simulink model "View_Speed"  (R2024b)
settings: Solver=FixedStepDiscrete  StartTime=0.0  StopTime=10.0  FixedStep=0.1  RelTol=1e-3  EnableMultiTasking=on
values from neighbouring files (symbols this model uses):
  C_BLANK = mpt.Parameter    [View_Speed_dd.m]
  C_CANADA = mpt.Parameter    [View_Speed_dd.m]
  C_DEFAULT_TOLER_A_VALUE = mpt.Parameter    [View_Speed_dd.m]
  C_DEFAULT_TOLER_B_VALUE = mpt.Parameter    [View_Speed_dd.m]
  C_MET_SPD_MAX_VALUE = mpt.Parameter    [View_Speed_dd.m]
  C_MET_SPD_MIN_THRESHOLD = mpt.Parameter    [View_Speed_dd.m]
  C_MEXICO = mpt.Parameter    [View_Speed_dd.m]
  C_SPEED_1KMPH = mpt.Parameter    [View_Speed_dd.m]
  C_SPEED_2KMPH = mpt.Parameter    [View_Speed_dd.m]
  C_SPEED_ZERO = mpt.Parameter    [View_Speed_dd.m]
  C_USA = mpt.Parameter    [View_Speed_dd.m]
  cFACTOR = mpt.Parameter    [View_Speed_dd.m]
  cOFFSET = mpt.Parameter    [View_Speed_dd.m]
  eTOLER_AOut = mpt.Parameter    [View_Speed_dd.m]
  eTOLER_BOut = mpt.Parameter    [View_Speed_dd.m]
  IGN_TRAN_TIMER_MS = mpt.Parameter    [View_Speed_dd.m]
  RESOLUTION_100 = mpt.Parameter    [View_Speed_dd.m]
  RTE_E_MAX_AGE_EXCEEDED = mpt.Parameter    [View_Speed_rte_types.m]
  RTE_E_NEVER_RECEIVED = mpt.Parameter    [View_Speed_rte_types.m]
  VAL_ONE = mpt.Parameter    [View_Speed_dd.m]
  View_Speed_cTaskPeriod = mpt.Parameter    [View_Speed_rte_types.m]
undefined symbols (not defined in the file or in its folder): Arr_u8_100_type_instance, Arr_u8_1024_type_instance, Arr_u8_10_type_instance, Arr_u8_128_type_instance, Arr_u8_16_type_instance, Arr_u8_17_type_instance, Arr_u8_2048_type_instance, Arr_u8_256_type_instance, Arr_u8_32_type_instance, Arr_u8_3_type_instance, Arr_u8_46_type_instance, Arr_u8_48_type_instance, Arr_u8_61_type_instance, Arr_u8_64_type_instance, Arr_u8_8_type_instance, Arr_u8_9_type_instance, CLUSTER_INACTIVE, eMET_SPDOut, eSP_ADR, eSP_CANADA, eSP_ECE, eSP_EUROPE, eSP_KOREA_FMVSS, eSP_KOREA_UN_R, eSP_MEXICO_FMVSS, eSP_MEXICO_UN_R, eSP_UK, eSP_USA, eVehicleSpeedABSIn, IgnOff, IgnOn, pJustRcvdStatus, RxCan_SignalClearJustRcvdStatus, RxCan_SignalGetJustRcvdStatus, RxCan_SignalInvalidProcessingControl, RxCan_SignalMissingProcessingControl, RxCan_SignalNRProcessingControl, SignalId, Status, tRxSignalId_type_instance, tRxSignalJustRcvdStatus_type_instance, tRxSignalStatus_type_instance, tTxSigConfirmStatus_type_instance, tTxSignalId_type_instance, TxCan_ClearCanSignalTxConfirmation
libraries: simulink x8
(part 2 of 2)

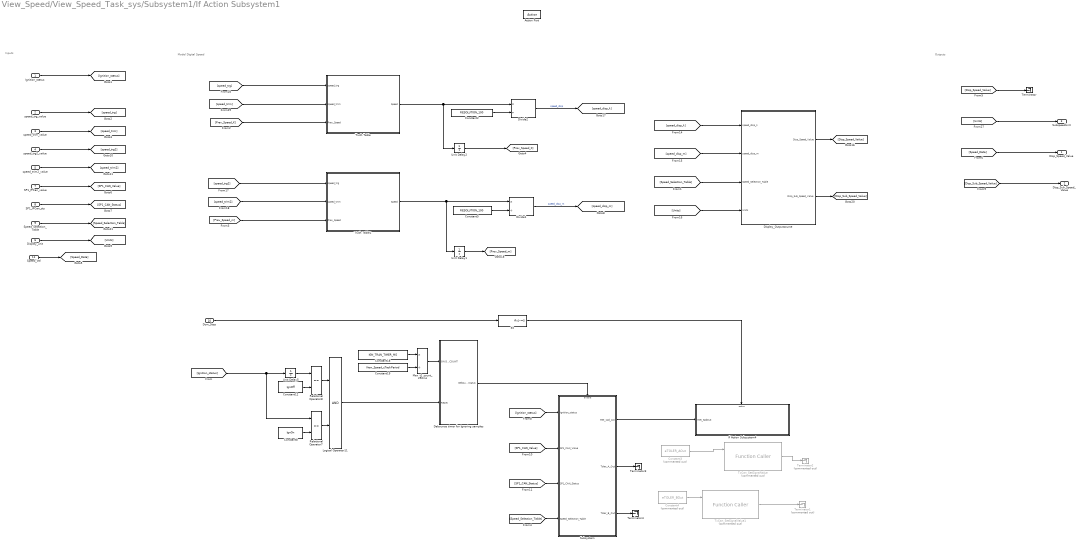
== system View_Speed/View_Speed_Task_sys/Subsystem1/If Action Subsystem1 ==
  note: Model Digital Speed
  note: Outputs
  note: Inputs
  Ignition_status : Inport  OutDataTypeStr=IgntionSubstateType
  speed_trg_value : Inport  Port=2  OutDataTypeStr=uint16
  speed_trim_value : Inport  Port=3  OutDataTypeStr=uint16
  speed_trg2_value : Inport  Port=4  OutDataTypeStr=uint16
  speed_trim2_value : Inport  Port=5  OutDataTypeStr=uint16
  Display_unit : Inport  Port=6  OutDataTypeStr=uint8
  SP1_IPCan_value : Inport  Port=7  OutDataTypeStr=uint16
  SP1_IPCan_sts : Inport  Port=8  OutDataTypeStr=uint8
  Speed_Selection_Table : Inport  Port=9  OutDataTypeStr=uint8
  Dcm_Stop : Inport  Port=10
  Speed_Val : Inport  Port=11  OutDataTypeStr=uint16
  Action Port : ActionPort  ActionPortLabel=if(u1 ~= u2)
  Constant12 : Constant  Value=IgnOff  OutDataTypeStr=uint8
  Constant18 : Constant  Value=IGN_TRAN_TIMER_MS  OutDataTypeStr=uint16
  Constant19 : Constant  Value=View_Speed_cTaskPeriod
  Constant2 : Constant  Value=RESOLUTION_100  OutDataTypeStr=uint16
  Constant3 : Constant  Commented=on  Value=eTOLER_AOut  OutDataTypeStr=uint8
  Constant4 : Constant  Commented=on  Value=eTOLER_BOut  OutDataTypeStr=uint8
  Constant5 : Constant  Value=RESOLUTION_100  OutDataTypeStr=uint16
  Constant8 : Constant  Value=IgnOn  OutDataTypeStr=uint8
  Debounce timer for Ignoring samples : Subsystem  TreatAsAtomicUnit=on
  Display_Outputsource : Subsystem
  Divide1 : Product  Inputs=*/
  Divide2 : Product  Inputs=*/
  If Action Subsystem4 : Subsystem  TreatAsAtomicUnit=on
  If2 : If  IfExpression=u1~=1  ShowElse=off
  Logical Operator11 : Logic  AllPortsSameDT=off  OutDataTypeStr=boolean
  Max_t1_count_250ms : Product  Inputs=*/  OutDataTypeStr=uint16
  Relational Operator7 : RelationalOperator  Operator===  OutDataTypeStr=boolean  InputSameDT=off
  Relational Operator8 : RelationalOperator  Operator===  OutDataTypeStr=boolean  InputSameDT=off
  Subsystem : Subsystem
  Terminator : Terminator
  Terminator1 : Terminator  Commented=on
  Terminator2 : Terminator  Commented=on
  Terminator3 : Terminator
  Terminator4 : Terminator
  Truth Table : Truth Table  TreatAsAtomicUnit=on  RTWFcnName=Speed_Value_Update
      settings: RTWSystemCode=Reusable function  RTWFcnNameOpts=User specified
  Truth Table1 : Truth Table  TreatAsAtomicUnit=on  RTWFcnName=Speed_Value_Update
      settings: RTWSystemCode=Reusable function  RTWFcnNameOpts=User specified
  TxCan_SetSignalValue : FunctionCaller  Commented=on  FunctionPrototype=error_status = TxCan_SetSignalValue(SignalId,pTxSignalData)  InputArgumentSpecifications=tTxSignalId_type_instance(1) ,uint8(1)  OutputArgumentSpecifications=uint8(1)
  TxCan_SetSignalValue1 : FunctionCaller  Commented=on  FunctionPrototype=error_status = TxCan_SetSignalValue(SignalId,pTxSignalData)  InputArgumentSpecifications=tTxSignalId_type_instance(1) ,uint8(1)  OutputArgumentSpecifications=uint8(1)
  Unit Delay1 : UnitDelay  SampleTime=-1  StateName=Prev_Speed_m  HasFrameUpgradeWarning=on
  Unit Delay2 : UnitDelay  SampleTime=-1  StateName=Prev_Speed_k  HasFrameUpgradeWarning=on
  Unit Delay5 : UnitDelay  SampleTime=-1  StateName=PrevWUSIgnState1  HasFrameUpgradeWarning=on
  Disp_Speed_Value : Outport  VectorParamsAs1DForOutWhenUnconnected=off
  Disp_Sub_Speed_Value : Outport  Port=2  VectorParamsAs1DForOutWhenUnconnected=off
  SubspeedUnit : Outport  Port=3  VectorParamsAs1DForOutWhenUnconnected=off
  wires:
  speed_trg2_value/1 -> [speed_trg2]
  SP1_IPCan_sts/1 -> [SP1_CAN_Status]
  Debounce timer for Ignoring samples/1(Debounced SW status) -> Subsystem/Enable
  speed_trim_value/1 -> [speed_trim]
  Ignition_status/1 -> [Ignition_status]
  Logical Operator11/1 -> Debounce timer for Ignoring samples/2("Reset ")
  Unit Delay5/1 -> Relational Operator8/1
  If2/1 -> If Action Subsystem4/Action
  Constant5/1 -> Divide1/2
  Max_t1_count_250ms/1 -> Debounce timer for Ignoring samples/1(ON DBNC COUNT)
  Constant12/1 -> Relational Operator8/2
  Constant18/1 -> Max_t1_count_250ms/1
  [Ignition_status] -> Subsystem/1(Ignition_status)
  [Ignition_status] -> Unit Delay5/1, Relational Operator7/1
  speed_trg_value/1 -> [speed_trg]
  [speed_disp_m] -> Display_Outputsource/2(speed_disp_m)
  Truth Table1/1(Speed) -> Unit Delay1/1, Divide1/1
  Display_unit/1 -> [Units]
  Constant19/1 -> Max_t1_count_250ms/2
  Subsystem/1(Met_spd_out) -> If Action Subsystem4/1(Met_SpdOut)
  [SP1_CAN_Value] -> Subsystem/2(SP1_CAN_Value)
  [SP1_CAN_Status] -> Subsystem/3(SP1_CAN_Status)
  Dcm_Stop/1 -> If2/1
  [speed_disp_k] -> Display_Outputsource/1(speed_disp_k)
  Relational Operator8/1 -> Logical Operator11/1
  Relational Operator7/1 -> Logical Operator11/2
  [Units] -> Display_Outputsource/4(Units)
  Constant3/1 -> TxCan_SetSignalValue/1
  Divide1/1 -> [speed_disp_m]  "speed_disp_m"
  Constant8/1 -> Relational Operator7/2
  SP1_IPCan_value/1 -> [SP1_CAN_Value]
  speed_trim2_value/1 -> [speed_trim2]
  Constant4/1 -> TxCan_SetSignalValue1/1
  [Units] -> SubspeedUnit/1
  [speed_trg] -> Truth Table/1(speed_trg)
  [speed_trim] -> Truth Table/2(speed_trim)
  Divide2/1 -> [speed_disp_k]  "speed_disp"
  Truth Table/1(Speed) -> Divide2/1, Unit Delay2/1
  Constant2/1 -> Divide2/2
  Unit Delay2/1 -> [Prev_Speed_K]
  [Prev_Speed_K] -> Truth Table/3(Prev_Speed)
  [speed_trg2] -> Truth Table1/1(speed_trg)
  [speed_trim2] -> Truth Table1/2(speed_trim)
  Unit Delay1/1 -> [Prev_Speed_m]
  [Prev_Speed_m] -> Truth Table1/3(Prev_Speed)
  Display_Outputsource/1(Disp_Speed_Value) -> [Disp_Speed_Value]
  Display_Outputsource/2(Disp_Sub_Speed_Value) -> [Disp_Sub_Speed_Value]
  [Speed_Data] -> Disp_Speed_Value/1
  [Disp_Sub_Speed_Value] -> Disp_Sub_Speed_Value/1
  Speed_Selection_Table/1 -> [Speed_Selection_Table]
  [Speed_Selection_Table] -> Display_Outputsource/3(Speed_Selection_Table)
  [Speed_Selection_Table] -> Subsystem/4(Speed_Selection_Table)
  Speed_Val/1 -> [Speed_Data]
  [Disp_Speed_Value] -> Terminator/1
  TxCan_SetSignalValue1/1 -> Terminator1/1
  TxCan_SetSignalValue/1 -> Terminator2/1
  Subsystem/2(Toler_A_Out) -> Terminator3/1
  Subsystem/3(Toler_B_Out) -> Terminator4/1

== system View_Speed/View_Speed_Task_sys/Subsystem1/If Action Subsystem1/Debounce timer for Ignoring samples ==
  note: 1. When Reset input is FALSE, allow counter to increment.
      |        (Limit to MAX when MAX count is reached)
  ON DBNC COUNT : Inport  OutDataTypeStr=uint16
  "Reset " : Inport  Port=2  OutDataTypeStr=boolean
  Constant1 : Constant  OutDataTypeStr=uint8
  Constant2 : Constant  Value=0  OutDataTypeStr=uint8
  Constant7 : Constant  Value=0  OutDataTypeStr=uint8
  Relational Operator1 : RelationalOperator  Operator=~=  OutDataTypeStr=boolean  InputSameDT=off
  Relational Operator4 : RelationalOperator  OutDataTypeStr=boolean  InputSameDT=off
  Sum : Sum  Inputs=|++
  Switch2 : Switch  Criteria=u2 ~= 0  OutDataTypeStr=uint32  SaturateOnIntegerOverflow=off  InputSameDT=off
  Switch3 : Switch  Criteria=u2 ~= 0  OutDataTypeStr=uint32  SaturateOnIntegerOverflow=off  InputSameDT=off
  Unit Delay2 : UnitDelay  SampleTime=-1  StateName=Igntran_timer_count  HasFrameUpgradeWarning=on
  Debounced SW status : Outport  VectorParamsAs1DForOutWhenUnconnected=off
  wires:
  "Reset "/1 -> Relational Operator1/2
  Constant7/1 -> Relational Operator1/1
  Relational Operator1/1 -> Switch2/2
  Switch2/1 -> Switch3/3, Relational Operator4/1
  ON DBNC COUNT/1 -> Relational Operator4/2, Switch3/1
  Switch3/1 -> Unit Delay2/1
  Constant2/1 -> Switch2/1
  Sum/1 -> Switch2/3
  Unit Delay2/1 -> Sum/2
  Constant1/1 -> Sum/1
  Relational Operator4/1 -> Debounced SW status/1, Switch3/2

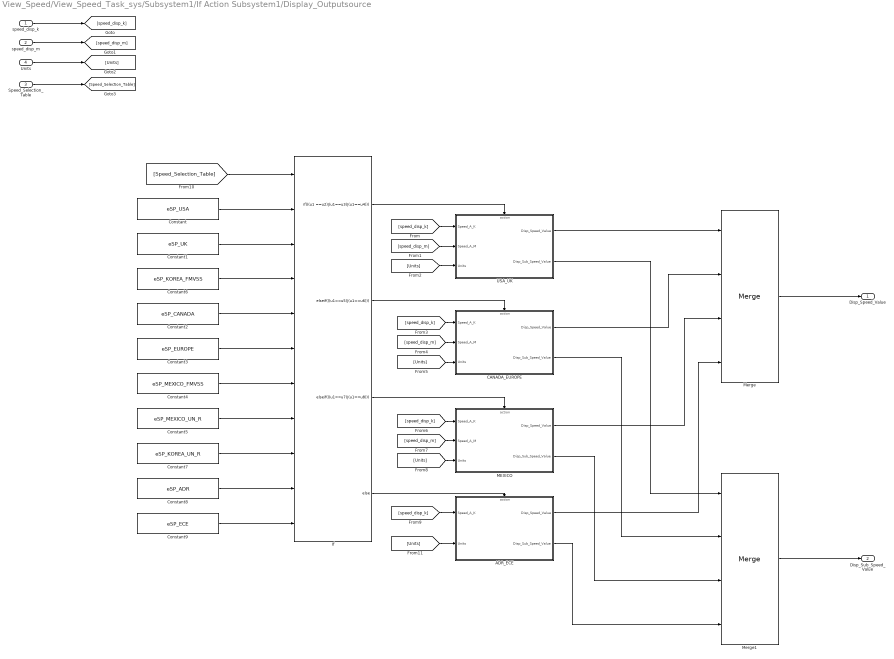
== system View_Speed/View_Speed_Task_sys/Subsystem1/If Action Subsystem1/Display_Outputsource ==
  speed_disp_k : Inport
  speed_disp_m : Inport  Port=2
  Speed_Selection_Table : Inport  Port=3
  Units : Inport  Port=4
  ADR_ECE : Subsystem  TreatAsAtomicUnit=on
  CANADA_EUROPE : Subsystem  TreatAsAtomicUnit=on
  Constant : Constant  Value=eSP_USA  OutDataTypeStr=uint8
  Constant1 : Constant  Value=eSP_UK  OutDataTypeStr=uint8
  Constant2 : Constant  Value=eSP_CANADA  OutDataTypeStr=uint8
  Constant3 : Constant  Value=eSP_EUROPE  OutDataTypeStr=uint8
  Constant4 : Constant  Value=eSP_MEXICO_FMVSS  OutDataTypeStr=uint8
  Constant5 : Constant  Value=eSP_MEXICO_UN_R  OutDataTypeStr=uint8
  Constant6 : Constant  Value=eSP_KOREA_FMVSS  OutDataTypeStr=uint8
  Constant7 : Constant  Value=eSP_KOREA_UN_R  OutDataTypeStr=uint8
  Constant8 : Constant  Value=eSP_ADR  OutDataTypeStr=uint8
  Constant9 : Constant  Value=eSP_ECE  OutDataTypeStr=uint8
  If : If  NumInputs=11  IfExpression=((u1 ==u2)|(u1==u3)|(u1==u4))  ElseIfExpressions=((u1==u5)|(u1==u6)),((u1==u7)|(u1==u8))
  MEXICO : Subsystem  TreatAsAtomicUnit=on
  Merge : Merge  Inputs=4
  Merge1 : Merge  Inputs=4
  USA_UK : Subsystem  TreatAsAtomicUnit=on
  Disp_Speed_Value : Outport  VectorParamsAs1DForOutWhenUnconnected=off
  Disp_Sub_Speed_Value : Outport  Port=2  VectorParamsAs1DForOutWhenUnconnected=off
  wires:
  MEXICO/1(Disp_Speed_Value) -> Merge/3
  If/3 -> MEXICO/Action
  If/2 -> CANADA_EUROPE/Action
  Merge/1 -> Disp_Speed_Value/1
  USA_UK/1(Disp_Speed_Value) -> Merge/1
  If/1 -> USA_UK/Action
  CANADA_EUROPE/1(Disp_Speed_Value) -> Merge/2
  If/4 -> ADR_ECE/Action
  ADR_ECE/1(Disp_Speed_Value) -> Merge/4
  USA_UK/2(Disp_Sub_Speed_Value) -> Merge1/1
  CANADA_EUROPE/2(Disp_Sub_Speed_Value) -> Merge1/2
  MEXICO/2(Disp_Sub_Speed_Value) -> Merge1/3
  ADR_ECE/2(Disp_Sub_Speed_Value) -> Merge1/4
  Merge1/1 -> Disp_Sub_Speed_Value/1
  speed_disp_k/1 -> [speed_disp_k]
  speed_disp_m/1 -> [speed_disp_m]
  Units/1 -> [Units]
  [speed_disp_k] -> USA_UK/1(Speed_A_K)
  [speed_disp_m] -> USA_UK/2(Speed_A_M)
  [Units] -> USA_UK/3(Units)
  [speed_disp_k] -> CANADA_EUROPE/1(Speed_A_K)
  [speed_disp_m] -> CANADA_EUROPE/2(Speed_A_M)
  [Units] -> CANADA_EUROPE/3(Units)
  [speed_disp_k] -> MEXICO/1(Speed_A_K)
  [speed_disp_m] -> MEXICO/2(Speed_A_M)
  [Units] -> MEXICO/3(Units)
  [speed_disp_k] -> ADR_ECE/1(Speed_A_K)
  [Units] -> ADR_ECE/2(Units)
  Speed_Selection_Table/1 -> [Speed_Selection_Table]
  [Speed_Selection_Table] -> If/1
  Constant/1 -> If/2
  Constant1/1 -> If/3
  Constant6/1 -> If/4
  Constant2/1 -> If/5
  Constant3/1 -> If/6
  Constant4/1 -> If/7
  Constant5/1 -> If/8
  Constant7/1 -> If/9
  Constant8/1 -> If/10
  Constant9/1 -> If/11

== system View_Speed/View_Speed_Task_sys/Subsystem1/If Action Subsystem1/If Action Subsystem4 ==
  Met_SpdOut : Inport  OutDataTypeStr=uint8
  Action Port : ActionPort  ActionPortLabel=if(u1~=1)
  Constant2 : Constant  Commented=on  Value=eMET_SPDOut  OutDataTypeStr=uint16
  Terminator : Terminator  Commented=on
  TxCanAdapterTx_SetSignalValueU8 : FunctionCaller  Commented=on  FunctionPrototype=error_status = TxCanAdapterTx_SetSignalValueU8(SignalId,pTxSignalData)  InputArgumentSpecifications=tTxSignalId_type_instance(1) ,uint8(1)  OutputArgumentSpecifications=uint8(1)
  wires:
  Met_SpdOut/1 -> TxCanAdapterTx_SetSignalValueU8/2
  TxCanAdapterTx_SetSignalValueU8/1 -> Terminator/1
  Constant2/1 -> TxCanAdapterTx_SetSignalValueU8/1

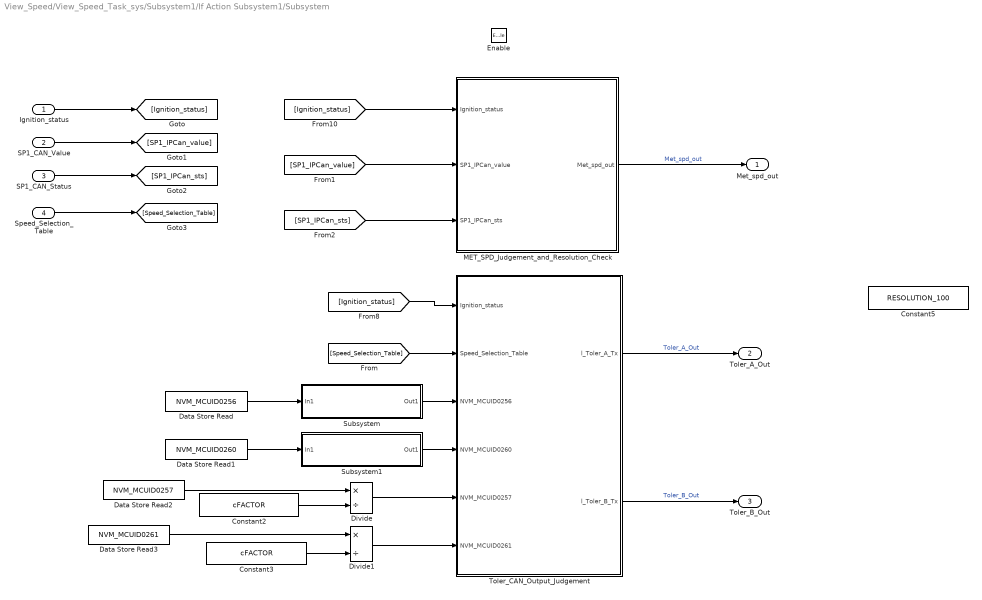
== system View_Speed/View_Speed_Task_sys/Subsystem1/If Action Subsystem1/Subsystem ==
  Ignition_status : Inport
  SP1_CAN_Value : Inport  Port=2
  SP1_CAN_Status : Inport  Port=3
  Speed_Selection_Table : Inport  Port=4
  Enable : EnablePort
  Constant2 : Constant  Value=cFACTOR  OutDataTypeStr=uint16
  Constant3 : Constant  Value=cFACTOR  OutDataTypeStr=uint16
  Constant5 : Constant  Value=RESOLUTION_100  OutDataTypeStr=uint16
  Data Store Read : DataStoreRead  DataStoreName=NVM_MCUID0256  IndexOptions=Index vector (dialog)  Indices=1  OutputSizes=1
  Data Store Read1 : DataStoreRead  DataStoreName=NVM_MCUID0260  IndexOptions=Index vector (dialog)  Indices=1  OutputSizes=1
  Data Store Read2 : DataStoreRead  DataStoreName=NVM_MCUID0257  IndexOptions=Index vector (dialog)  Indices=1  OutputSizes=1
  Data Store Read3 : DataStoreRead  DataStoreName=NVM_MCUID0261  IndexOptions=Index vector (dialog)  Indices=1  OutputSizes=1
  Divide : Product  Inputs=*/  OutDataTypeStr=uint8
  Divide1 : Product  Inputs=*/  OutDataTypeStr=uint8
  MET_SPD_Judgement_and_Resolution_Check : Subsystem
  Subsystem : Subsystem  RTWFileName=Resolution_Handling
      settings: RTWFileNameOpts=User specified
  Subsystem1 : Subsystem  RTWFileName=Resolution_Handling
      settings: RTWFileNameOpts=User specified
  Toler_CAN_Output_Judgement : Truth Table  TreatAsAtomicUnit=on
  Met_spd_out : Outport  OutDataTypeStr=uint8  VectorParamsAs1DForOutWhenUnconnected=off
  Toler_A_Out : Outport  Port=2  OutDataTypeStr=uint8  VectorParamsAs1DForOutWhenUnconnected=off
  Toler_B_Out : Outport  Port=3  OutDataTypeStr=uint8  VectorParamsAs1DForOutWhenUnconnected=off
  wires:
  Toler_CAN_Output_Judgement/2(l_Toler_B_Tx) -> Toler_B_Out/1  "Toler_B_Out"
  Toler_CAN_Output_Judgement/1(l_Toler_A_Tx) -> Toler_A_Out/1  "Toler_A_Out"
  [SP1_IPCan_sts] -> MET_SPD_Judgement_and_Resolution_Check/3(SP1_IPCan_sts)
  [SP1_IPCan_value] -> MET_SPD_Judgement_and_Resolution_Check/2(SP1_IPCan_value)
  [Ignition_status] -> Toler_CAN_Output_Judgement/1(Ignition_status)
  MET_SPD_Judgement_and_Resolution_Check/1(Met_spd_out) -> Met_spd_out/1  "Met_spd_out"
  [Ignition_status] -> MET_SPD_Judgement_and_Resolution_Check/1(Ignition_status)
  Ignition_status/1 -> [Ignition_status]
  SP1_CAN_Value/1 -> [SP1_IPCan_value]
  SP1_CAN_Status/1 -> [SP1_IPCan_sts]
  Speed_Selection_Table/1 -> [Speed_Selection_Table]
  Data Store Read1/1 -> Subsystem1/1(In1)
  Data Store Read2/1 -> Divide/1
  [Speed_Selection_Table] -> Toler_CAN_Output_Judgement/2(Speed_Selection_Table)
  Data Store Read/1 -> Subsystem/1(In1)
  Subsystem/1(Out1) -> Toler_CAN_Output_Judgement/3(NVM_MCUID0256)
  Subsystem1/1(Out1) -> Toler_CAN_Output_Judgement/4(NVM_MCUID0260)
  Divide/1 -> Toler_CAN_Output_Judgement/5(NVM_MCUID0257)
  Divide1/1 -> Toler_CAN_Output_Judgement/6(NVM_MCUID0261)
  Constant2/1 -> Divide/2
  Data Store Read3/1 -> Divide1/1
  Constant3/1 -> Divide1/2

== system View_Speed/View_Speed_Task_sys/Subsystem1/If Action Subsystem1/Display_Outputsource/ADR_ECE ==
  Speed_A_K : Inport
  Units : Inport  Port=2
  Action Port : ActionPort  ActionPortLabel=else
  If : If  IfExpression=u1 == 0
  If Action Subsystem : Subsystem  TreatAsAtomicUnit=on
  If Action Subsystem1 : Subsystem  TreatAsAtomicUnit=on
  Merge : Merge
  Merge1 : Merge
  Disp_Speed_Value : Outport  VectorParamsAs1DForOutWhenUnconnected=off
  Disp_Sub_Speed_Value : Outport  Port=2  VectorParamsAs1DForOutWhenUnconnected=off
  wires:
  If/2 -> If Action Subsystem1/Action
  Merge/1 -> Disp_Speed_Value/1  "Disp_Speed_Value"
  Merge1/1 -> Disp_Sub_Speed_Value/1  "Disp_Sub_Speed_Value"
  If Action Subsystem/1(Disp_Speed) -> Merge/1
  Units/1 -> If/1
  If/1 -> If Action Subsystem/Action
  If Action Subsystem1/2(Disp_Sub_Speed) -> Merge1/2
  If Action Subsystem/2(Disp_Sub_Speed) -> Merge1/1
  If Action Subsystem1/1(Disp_Speed) -> Merge/2
  Speed_A_K/1 -> If Action Subsystem/1(Speed_A_K)

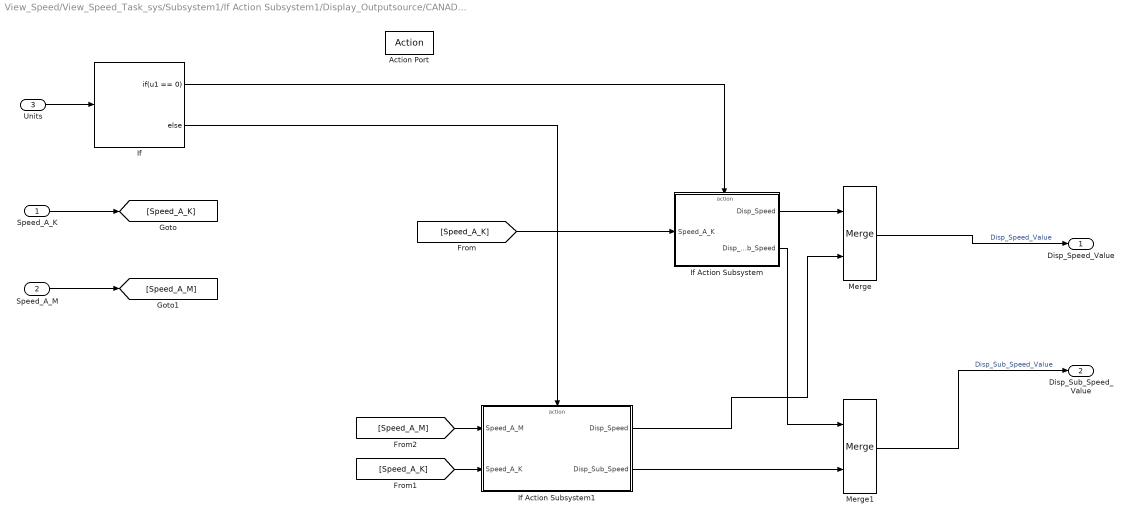
== system View_Speed/View_Speed_Task_sys/Subsystem1/If Action Subsystem1/Display_Outputsource/CANADA_EUROPE ==
  Speed_A_K : Inport
  Speed_A_M : Inport  Port=2
  Units : Inport  Port=3
  Action Port : ActionPort  ActionPortLabel=elseif(((u1==u5)|(u1==u6)))
  If : If  IfExpression=u1 == 0
  If Action Subsystem : Subsystem  TreatAsAtomicUnit=on
  If Action Subsystem1 : Subsystem  TreatAsAtomicUnit=on
  Merge : Merge
  Merge1 : Merge
  Disp_Speed_Value : Outport  VectorParamsAs1DForOutWhenUnconnected=off
  Disp_Sub_Speed_Value : Outport  Port=2  VectorParamsAs1DForOutWhenUnconnected=off
  wires:
  If/2 -> If Action Subsystem1/Action
  If Action Subsystem/1(Disp_Speed) -> Merge/1
  If Action Subsystem1/2(Disp_Sub_Speed) -> Merge1/2
  If Action Subsystem/2(Disp_Sub_Speed) -> Merge1/1
  If Action Subsystem1/1(Disp_Speed) -> Merge/2
  If/1 -> If Action Subsystem/Action
  Merge1/1 -> Disp_Sub_Speed_Value/1  "Disp_Sub_Speed_Value"
  Units/1 -> If/1
  Merge/1 -> Disp_Speed_Value/1  "Disp_Speed_Value"
  Speed_A_M/1 -> [Speed_A_M]
  Speed_A_K/1 -> [Speed_A_K]
  [Speed_A_K] -> If Action Subsystem/1(Speed_A_K)
  [Speed_A_K] -> If Action Subsystem1/2(Speed_A_K)
  [Speed_A_M] -> If Action Subsystem1/1(Speed_A_M)

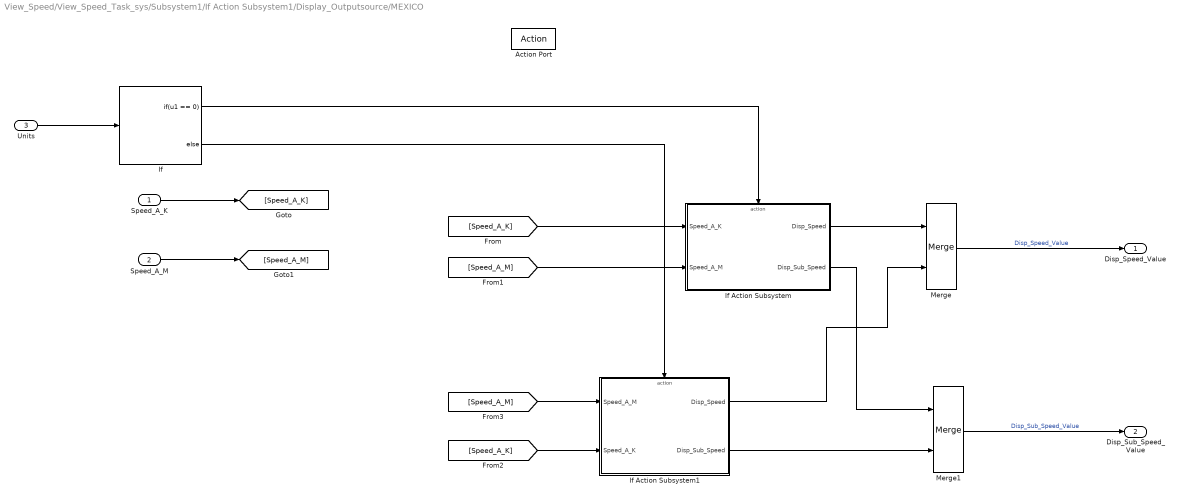
== system View_Speed/View_Speed_Task_sys/Subsystem1/If Action Subsystem1/Display_Outputsource/MEXICO ==
  Speed_A_K : Inport
  Speed_A_M : Inport  Port=2
  Units : Inport  Port=3
  Action Port : ActionPort  ActionPortLabel=elseif(((u1==u7)|(u1==u8)))
  If : If  IfExpression=u1 == 0
  If Action Subsystem : Subsystem  TreatAsAtomicUnit=on
  If Action Subsystem1 : Subsystem  TreatAsAtomicUnit=on
  Merge : Merge
  Merge1 : Merge
  Disp_Speed_Value : Outport  VectorParamsAs1DForOutWhenUnconnected=off
  Disp_Sub_Speed_Value : Outport  Port=2  VectorParamsAs1DForOutWhenUnconnected=off
  wires:
  If/2 -> If Action Subsystem1/Action
  Merge/1 -> Disp_Speed_Value/1  "Disp_Speed_Value"
  Merge1/1 -> Disp_Sub_Speed_Value/1  "Disp_Sub_Speed_Value"
  If Action Subsystem/1(Disp_Speed) -> Merge/1
  Units/1 -> If/1
  If/1 -> If Action Subsystem/Action
  If Action Subsystem1/2(Disp_Sub_Speed) -> Merge1/2
  If Action Subsystem/2(Disp_Sub_Speed) -> Merge1/1
  If Action Subsystem1/1(Disp_Speed) -> Merge/2
  Speed_A_K/1 -> [Speed_A_K]
  Speed_A_M/1 -> [Speed_A_M]
  [Speed_A_K] -> If Action Subsystem/1(Speed_A_K)
  [Speed_A_M] -> If Action Subsystem/2(Speed_A_M)
  [Speed_A_M] -> If Action Subsystem1/1(Speed_A_M)
  [Speed_A_K] -> If Action Subsystem1/2(Speed_A_K)

== system View_Speed/View_Speed_Task_sys/Subsystem1/If Action Subsystem1/Display_Outputsource/USA_UK ==
  Speed_A_K : Inport
  Speed_A_M : Inport  Port=2
  Units : Inport  Port=3
  Action Port : ActionPort  ActionPortLabel=if(((u1 ==u2)|(u1==u3)|(u1==u4)))
  If : If  IfExpression=u1 == 0
  If Action Subsystem : Subsystem  TreatAsAtomicUnit=on
  If Action Subsystem1 : Subsystem  TreatAsAtomicUnit=on
  Merge : Merge
  Merge1 : Merge
  Disp_Speed_Value : Outport  VectorParamsAs1DForOutWhenUnconnected=off
  Disp_Sub_Speed_Value : Outport  Port=2  VectorParamsAs1DForOutWhenUnconnected=off
  wires:
  Merge/1 -> Disp_Speed_Value/1  "Disp_Speed_Value"
  Units/1 -> If/1
  If/1 -> If Action Subsystem/Action
  If/2 -> If Action Subsystem1/Action
  If Action Subsystem/1(Disp_Speed) -> Merge/1
  If Action Subsystem1/1(Disp_Speed) -> Merge/2
  If Action Subsystem/2(Disp_Sub_Speed) -> Merge1/1
  Merge1/1 -> Disp_Sub_Speed_Value/1  "Disp_Sub_Speed_Value"
  If Action Subsystem1/2(Disp_Sub_Speed) -> Merge1/2
  Speed_A_K/1 -> [Speed_A_K]
  Speed_A_M/1 -> [Speed_A_M]
  [Speed_A_K] -> If Action Subsystem/1(Speed_A_K)
  [Speed_A_M] -> If Action Subsystem/2(Speed_A_M)
  [Speed_A_M] -> If Action Subsystem1/1(Speed_A_M)

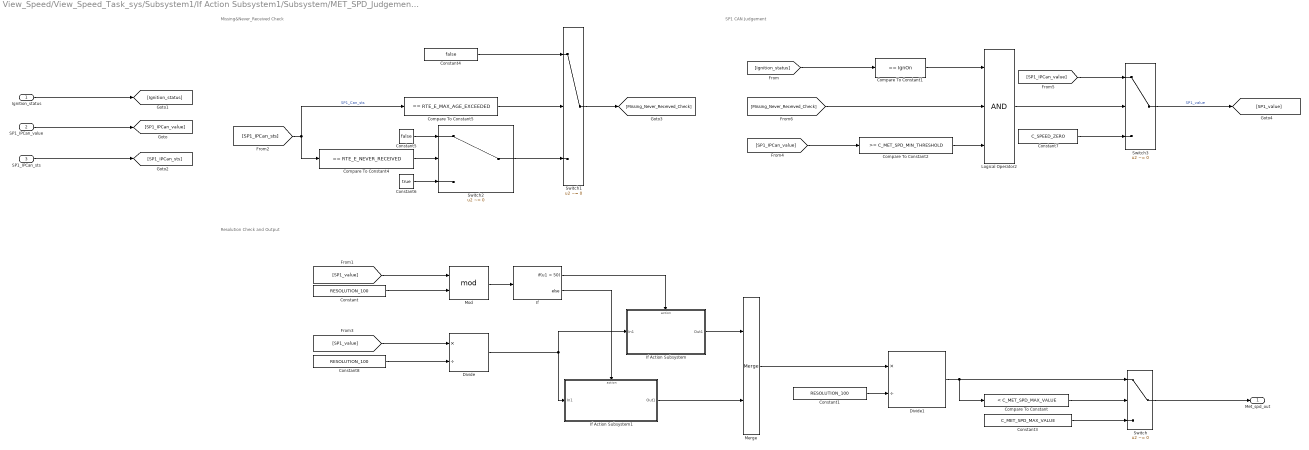
== system View_Speed/View_Speed_Task_sys/Subsystem1/If Action Subsystem1/Subsystem/MET_SPD_Judgement_and_Resolution_Check ==
  note: Resolution Check and Output
  note: SP1 CAN Judgement
  note: Missing&Never_Received Check
  Ignition_status : Inport  OutDataTypeStr=uint8
  SP1_IPCan_value : Inport  Port=2  OutDataTypeStr=uint16
  SP1_IPCan_sts : Inport  Port=3  OutDataTypeStr=uint8
  Compare To Constant : simulink/Logic and Bit Operations/Compare To Constant  relop=<  const=C_MET_SPD_MAX_VALUE  OutDataTypeStr=boolean
  Compare To Constant1 : simulink/Logic and Bit Operations/Compare To Constant  relop===  const=IgnOn  OutDataTypeStr=boolean
  Compare To Constant2 : simulink/Logic and Bit Operations/Compare To Constant  relop=>=  const=C_MET_SPD_MIN_THRESHOLD  OutDataTypeStr=boolean
  Compare To Constant4 : simulink/Logic and Bit Operations/Compare To Constant  relop===  const=RTE_E_NEVER_RECEIVED  OutDataTypeStr=boolean
  Compare To Constant5 : simulink/Logic and Bit Operations/Compare To Constant  relop===  const=RTE_E_MAX_AGE_EXCEEDED  OutDataTypeStr=boolean
  Constant : Constant  Value=RESOLUTION_100  OutDataTypeStr=uint16
  Constant1 : Constant  Value=RESOLUTION_100  OutDataTypeStr=uint16
  Constant3 : Constant  Value=C_MET_SPD_MAX_VALUE  OutDataTypeStr=uint16
  Constant4 : Constant  Value=false  OutDataTypeStr=uint16
  Constant5 : Constant  Value=false  OutDataTypeStr=uint8
  Constant6 : Constant  Value=true  OutDataTypeStr=uint8
  Constant7 : Constant  Value=C_SPEED_ZERO  OutDataTypeStr=uint16
  Constant8 : Constant  Value=RESOLUTION_100  OutDataTypeStr=uint16
  Divide : Product  Inputs=*/  SaturateOnIntegerOverflow=on
  Divide1 : Product  Inputs=*/  OutDataTypeStr=uint16  SaturateOnIntegerOverflow=on
  If : If  IfExpression=u1 < 50
  If Action Subsystem : Subsystem  TreatAsAtomicUnit=on
  If Action Subsystem1 : Subsystem  TreatAsAtomicUnit=on
  Logical Operator2 : Logic  Inputs=3  AllPortsSameDT=off  OutDataTypeStr=boolean
  Merge : Merge
  Mod : Math  Operator=mod  SignedPower=on
  Switch : Switch  Criteria=u2 ~= 0  OutDataTypeStr=uint8  SaturateOnIntegerOverflow=off  InputSameDT=off
  Switch1 : Switch  Criteria=u2 ~= 0  SaturateOnIntegerOverflow=off  InputSameDT=off
  Switch2 : Switch  Criteria=u2 ~= 0  RndMeth=Simplest  SaturateOnIntegerOverflow=off  InputSameDT=off
  Switch3 : Switch  Criteria=u2 ~= 0  SaturateOnIntegerOverflow=off  InputSameDT=off
  Met_spd_out : Outport  OutDataTypeStr=uint8  VectorParamsAs1DForOutWhenUnconnected=off
  wires:
  Constant8/1 -> Divide/2
  If/2 -> If Action Subsystem1/Action
  [SP1_value] -> Mod/1
  Constant/1 -> Mod/2
  If Action Subsystem1/1(Out1) -> Merge/2
  If/1 -> If Action Subsystem/Action
  Merge/1 -> Divide1/1
  Divide/1 -> If Action Subsystem/1(In1), If Action Subsystem1/1(In1)
  If Action Subsystem/1(Out1) -> Merge/1
  [SP1_value] -> Divide/1
  Mod/1 -> If/1
  Constant1/1 -> Divide1/2
  Compare To Constant/1 -> Switch/2
  Constant3/1 -> Switch/3
  Switch/1 -> Met_spd_out/1
  Ignition_status/1 -> [Ignition_status]
  Divide1/1 -> Compare To Constant/1, Switch/1
  Compare To Constant5/1 -> Switch1/2
  Compare To Constant4/1 -> Switch2/2
  [SP1_IPCan_sts] -> Compare To Constant5/1, Compare To Constant4/1  "SP1_Can_sts"
  Constant5/1 -> Switch2/1
  [Ignition_status] -> Compare To Constant1/1
  Constant6/1 -> Switch2/3
  Switch2/1 -> Switch1/3
  Constant4/1 -> Switch1/1
  Compare To Constant1/1 -> Logical Operator2/1
  SP1_IPCan_value/1 -> [SP1_IPCan_value]
  SP1_IPCan_sts/1 -> [SP1_IPCan_sts]
  Constant7/1 -> Switch3/3
  Logical Operator2/1 -> Switch3/2
  Switch3/1 -> [SP1_value]  "SP1_value"
  [SP1_IPCan_value] -> Compare To Constant2/1
  Compare To Constant2/1 -> Logical Operator2/3
  Switch1/1 -> [Missing_Never_Received_Check]
  [Missing_Never_Received_Check] -> Logical Operator2/2
  [SP1_IPCan_value] -> Switch3/1

== system View_Speed/View_Speed_Task_sys/Subsystem1/If Action Subsystem1/Subsystem/Subsystem ==
  In1 : Inport
  Constant1 : Constant  Value=cOFFSET
  Constant2 : Constant  Value=cFACTOR  OutDataTypeStr=uint16
  Divide : Product  Inputs=*/  OutDataTypeStr=uint8
  Subtract : Sum  Inputs=+-  AccumDataTypeStr=uint16
  Out1 : Outport  OutDataTypeStr=uint8  VectorParamsAs1DForOutWhenUnconnected=off
  wires:
  Subtract/1 -> Divide/1
  Divide/1 -> Out1/1
  Constant2/1 -> Divide/2
  Constant1/1 -> Subtract/2
  In1/1 -> Subtract/1

== system View_Speed/View_Speed_Task_sys/Subsystem1/If Action Subsystem1/Subsystem/Subsystem1 ==
  In1 : Inport
  Constant1 : Constant  Value=cOFFSET
  Constant2 : Constant  Value=cFACTOR  OutDataTypeStr=uint16
  Divide : Product  Inputs=*/  OutDataTypeStr=uint8
  Subtract : Sum  Inputs=+-  AccumDataTypeStr=uint16
  Out1 : Outport  OutDataTypeStr=uint8  VectorParamsAs1DForOutWhenUnconnected=off
  wires:
  Subtract/1 -> Divide/1
  Divide/1 -> Out1/1
  Constant2/1 -> Divide/2
  Constant1/1 -> Subtract/2
  In1/1 -> Subtract/1

== system View_Speed/View_Speed_Task_sys/Subsystem1/If Action Subsystem1/Display_Outputsource/ADR_ECE/If Action Subsystem ==
  Speed_A_K : Inport
  Action Port : ActionPort  ActionPortLabel=if(u1 == 0)
  Constant1 : Constant  Value=C_BLANK
  Disp_Speed : Outport  VectorParamsAs1DForOutWhenUnconnected=off
  Disp_Sub_Speed : Outport  Port=2  VectorParamsAs1DForOutWhenUnconnected=off
  wires:
  Speed_A_K/1 -> Disp_Speed/1
  Constant1/1 -> Disp_Sub_Speed/1

== system View_Speed/View_Speed_Task_sys/Subsystem1/If Action Subsystem1/Display_Outputsource/ADR_ECE/If Action Subsystem1 ==
  Action Port : ActionPort  ActionPortLabel=else
  Constant : Constant  Value=C_BLANK
  Constant1 : Constant  Value=C_BLANK
  Disp_Speed : Outport  VectorParamsAs1DForOutWhenUnconnected=off
  Disp_Sub_Speed : Outport  Port=2  VectorParamsAs1DForOutWhenUnconnected=off
  wires:
  Constant/1 -> Disp_Speed/1
  Constant1/1 -> Disp_Sub_Speed/1

== system View_Speed/View_Speed_Task_sys/Subsystem1/If Action Subsystem1/Display_Outputsource/CANADA_EUROPE/If Action Subsystem ==
  Speed_A_K : Inport
  Action Port : ActionPort  ActionPortLabel=if(u1 == 0)
  Constant : Constant  Value=C_BLANK
  Disp_Speed : Outport  VectorParamsAs1DForOutWhenUnconnected=off
  Disp_Sub_Speed : Outport  Port=2  VectorParamsAs1DForOutWhenUnconnected=off
  wires:
  Speed_A_K/1 -> Disp_Speed/1
  Constant/1 -> Disp_Sub_Speed/1

== system View_Speed/View_Speed_Task_sys/Subsystem1/If Action Subsystem1/Display_Outputsource/CANADA_EUROPE/If Action Subsystem1 ==
  Speed_A_M : Inport
  Speed_A_K : Inport  Port=2
  Action Port : ActionPort  ActionPortLabel=else
  Disp_Speed : Outport  VectorParamsAs1DForOutWhenUnconnected=off
  Disp_Sub_Speed : Outport  Port=2  VectorParamsAs1DForOutWhenUnconnected=off
  wires:
  Speed_A_M/1 -> Disp_Speed/1
  Speed_A_K/1 -> Disp_Sub_Speed/1

== system View_Speed/View_Speed_Task_sys/Subsystem1/If Action Subsystem1/Display_Outputsource/MEXICO/If Action Subsystem ==
  Speed_A_K : Inport
  Speed_A_M : Inport  Port=2
  Action Port : ActionPort  ActionPortLabel=if(u1 == 0)
  Disp_Speed : Outport  VectorParamsAs1DForOutWhenUnconnected=off
  Disp_Sub_Speed : Outport  Port=2  VectorParamsAs1DForOutWhenUnconnected=off
  wires:
  Speed_A_K/1 -> Disp_Speed/1
  Speed_A_M/1 -> Disp_Sub_Speed/1

== system View_Speed/View_Speed_Task_sys/Subsystem1/If Action Subsystem1/Display_Outputsource/MEXICO/If Action Subsystem1 ==
  Speed_A_M : Inport
  Speed_A_K : Inport  Port=2
  Action Port : ActionPort  ActionPortLabel=else
  Disp_Speed : Outport  VectorParamsAs1DForOutWhenUnconnected=off
  Disp_Sub_Speed : Outport  Port=2  VectorParamsAs1DForOutWhenUnconnected=off
  wires:
  Speed_A_M/1 -> Disp_Speed/1
  Speed_A_K/1 -> Disp_Sub_Speed/1

== system View_Speed/View_Speed_Task_sys/Subsystem1/If Action Subsystem1/Display_Outputsource/USA_UK/If Action Subsystem ==
  Speed_A_K : Inport
  Speed_A_M : Inport  Port=2
  Action Port : ActionPort  ActionPortLabel=if(u1 == 0)
  Disp_Speed : Outport  VectorParamsAs1DForOutWhenUnconnected=off
  Disp_Sub_Speed : Outport  Port=2  VectorParamsAs1DForOutWhenUnconnected=off
  wires:
  Speed_A_K/1 -> Disp_Speed/1
  Speed_A_M/1 -> Disp_Sub_Speed/1

== system View_Speed/View_Speed_Task_sys/Subsystem1/If Action Subsystem1/Display_Outputsource/USA_UK/If Action Subsystem1 ==
  Speed_A_M : Inport
  Action Port : ActionPort  ActionPortLabel=else
  Constant : Constant  Value=C_BLANK
  Disp_Speed : Outport  VectorParamsAs1DForOutWhenUnconnected=off
  Disp_Sub_Speed : Outport  Port=2  VectorParamsAs1DForOutWhenUnconnected=off
  wires:
  Speed_A_M/1 -> Disp_Speed/1
  Constant/1 -> Disp_Sub_Speed/1

== system View_Speed/View_Speed_Task_sys/Subsystem1/If Action Subsystem1/Subsystem/MET_SPD_Judgement_and_Resolution_Check/If Action Subsystem ==
  In1 : Inport  OutDataTypeStr=uint16
  Action Port : ActionPort  ActionPortLabel=if(u1 < 50)
  Constant8 : Constant  Value=RESOLUTION_100  OutDataTypeStr=uint16
  Multiply : Product  OutDataTypeStr=uint16
  Out1 : Outport  OutDataTypeStr=uint16  VectorParamsAs1DForOutWhenUnconnected=off
  wires:
  In1/1 -> Multiply/1
  Constant8/1 -> Multiply/2
  Multiply/1 -> Out1/1

== system View_Speed/View_Speed_Task_sys/Subsystem1/If Action Subsystem1/Subsystem/MET_SPD_Judgement_and_Resolution_Check/If Action Subsystem1 ==
  In1 : Inport  OutDataTypeStr=uint16
  Action Port : ActionPort  ActionPortLabel=else
  Add : Sum  AccumDataTypeStr=int16
  Constant1 : Constant  Value=VAL_ONE
  Constant8 : Constant  Value=RESOLUTION_100  OutDataTypeStr=uint16
  Multiply : Product  OutDataTypeStr=uint16
  Out1 : Outport  OutDataTypeStr=uint16  VectorParamsAs1DForOutWhenUnconnected=off
  wires:
  Constant8/1 -> Multiply/2
  Constant1/1 -> Add/2
  In1/1 -> Add/1
  Add/1 -> Multiply/1
  Multiply/1 -> Out1/1

== matlab function View_Speed/View_Speed_Task_sys/Subsystem1/If Action Subsystem1/Subsystem/Toler_CAN_Output_Judgement ==
  data: l_Toler_A_Tx output uint8; Ignition_status input uint8; Speed_Selection_Table input; NVM_MCUID0256 input uint8; l_Toler_B_Tx output uint8; IgnOff parameter uint8; NVM_MCUID0260 input uint8; NVM_MCUID0257 input uint8; NVM_MCUID0261 input uint8; C_DEFAULT_TOLER_A_VALUE parameter uint8; C_DEFAULT_TOLER_B_VALUE parameter uint8; C_USA parameter; C_MEXICO parameter; C_CANADA parameter; eSP_CANADA parameter; eSP_USA parameter; eSP_MEXICO_FMVSS parameter; eSP_KOREA_FMVSS parameter
function [l_Toler_A_Tx, l_Toler_B_Tx] = fcn(Ignition_status, Speed_Selection_Table, NVM_MCUID0256, IgnOff, NVM_MCUID0260, NVM_MCUID0257, NVM_MCUID0261, C_DEFAULT_TOLER_A_VALUE, C_DEFAULT_TOLER_B_VALUE, C_USA, C_MEXICO, C_CANADA, eSP_CANADA, eSP_USA, eSP_MEXICO_FMVSS, eSP_KOREA_FMVSS)

aVarTruthTableCondition_1 = false;
aVarTruthTableCondition_2 = false;


% Ignition OFF

aVarTruthTableCondition_1 = logical(Ignition_status == IgnOff);

% Destination input US /CANADA/MEXICO

aVarTruthTableCondition_2 = logical(((Speed_Selection_Table == eSP_CANADA) || (Speed_Selection_Table == eSP_USA) || (Speed_Selection_Table == eSP_MEXICO_FMVSS) || (Speed_Selection_Table == eSP_KOREA_FMVSS)));

if (aVarTruthTableCondition_1)
    aFcnTruthTableAction_1();
elseif (aVarTruthTableCondition_2)
    aFcnTruthTableAction_2();
else % Default
    aFcnTruthTableAction_3();
end

function aFcnTruthTableAction_1()

% Ignition OFF case

l_Toler_A_Tx =C_DEFAULT_TOLER_A_VALUE;
l_Toler_B_Tx =C_DEFAULT_TOLER_B_VALUE;

function aFcnTruthTableAction_2()

% Destination input US /CANADA/MEXICO

l_Toler_A_Tx = NVM_MCUID0256;
l_Toler_B_Tx = NVM_MCUID0257;

function aFcnTruthTableAction_3()

% Destination input Other than US /CANADA/MEXICO

l_Toler_A_Tx =NVM_MCUID0260;
l_Toler_B_Tx =NVM_MCUID0261;

== matlab function View_Speed/View_Speed_Task_sys/Subsystem1/If Action Subsystem1/Truth Table ==
  data: speed_trg input; Speed output; speed_trim input; Prev_Speed input uint16; C_SPEED_1KMPH parameter; C_SPEED_2KMPH parameter; C_SPEED_ZERO parameter
function Speed = fcn(speed_trg, speed_trim, Prev_Speed, C_SPEED_1KMPH, C_SPEED_2KMPH, C_SPEED_ZERO)

aVarTruthTableCondition_1 = false;
aVarTruthTableCondition_2 = false;
aVarTruthTableCondition_3 = false;
aVarTruthTableCondition_4 = false;
aVarTruthTableCondition_5 = false;
aVarTruthTableCondition_6 = false;


% Speed trg greater than 2km/h

aVarTruthTableCondition_1 = logical((speed_trg > C_SPEED_2KMPH));

% Speed trg less than 2km/h and Prev Speed   greater than 2km/h

aVarTruthTableCondition_2 = logical((Prev_Speed >  C_SPEED_2KMPH));

% Speed trg less than 1km/h

aVarTruthTableCondition_3 = logical(((Prev_Speed ==  C_SPEED_2KMPH) && (speed_trg <=C_SPEED_1KMPH)));

% Speed trg is 2km/h  or Prev_Speed is less than 1km/h

aVarTruthTableCondition_4 = logical((Prev_Speed ==  C_SPEED_1KMPH) && ((speed_trg == C_SPEED_2KMPH) || (speed_trg == C_SPEED_ZERO)));

% Prev_Speed is 1km/h and Speed trim is 0

aVarTruthTableCondition_5 = logical(((Prev_Speed ==  C_SPEED_1KMPH) && (speed_trim == C_SPEED_ZERO)));

% pre Speed is 0km/h and Other Conditions

aVarTruthTableCondition_6 = logical((Prev_Speed ==  C_SPEED_ZERO) && ((speed_trg == C_SPEED_2KMPH) || (speed_trg == C_SPEED_1KMPH)));

if (aVarTruthTableCondition_1)
    aFcnTruthTableAction_1();
elseif (aVarTruthTableCondition_2)
    aFcnTruthTableAction_2();
elseif (aVarTruthTableCondition_3)
    aFcnTruthTableAction_3();
elseif (aVarTruthTableCondition_4)
    aFcnTruthTableAction_1();
elseif (aVarTruthTableCondition_5)
    aFcnTruthTableAction_4();
elseif (aVarTruthTableCondition_6)
    aFcnTruthTableAction_1();
else % Default
    aFcnTruthTableAction_5();
end

function aFcnTruthTableAction_1()

% Update Speed_k with Speed trigger

Speed = speed_trg;

function aFcnTruthTableAction_2()

% Update Speed_k with 2km/h

Speed = C_SPEED_2KMPH;

function aFcnTruthTableAction_3()

% Update Speed_k with 1km/h

Speed = C_SPEED_1KMPH;

function aFcnTruthTableAction_4()

% Update Speed_k with 0km/h

Speed = C_SPEED_ZERO;

function aFcnTruthTableAction_5()

% No Change

Speed = Prev_Speed;

== matlab function View_Speed/View_Speed_Task_sys/Subsystem1/If Action Subsystem1/Truth Table1 ==
  data: speed_trg input; Speed output; speed_trim input; Prev_Speed input uint16; C_SPEED_1KMPH parameter; C_SPEED_2KMPH parameter; C_SPEED_ZERO parameter
function Speed = fcn(speed_trg, speed_trim, Prev_Speed, C_SPEED_1KMPH, C_SPEED_2KMPH, C_SPEED_ZERO)

aVarTruthTableCondition_1 = false;
aVarTruthTableCondition_2 = false;
aVarTruthTableCondition_3 = false;
aVarTruthTableCondition_4 = false;
aVarTruthTableCondition_5 = false;
aVarTruthTableCondition_6 = false;


% Speed trg greater than 2km/h

aVarTruthTableCondition_1 = logical((speed_trg > C_SPEED_2KMPH));

% Speed trg less than 2km/h and Prev Speed   greater than 2km/h

aVarTruthTableCondition_2 = logical((Prev_Speed >  C_SPEED_2KMPH));

% Speed trg less than 1km/h

aVarTruthTableCondition_3 = logical(((Prev_Speed ==  C_SPEED_2KMPH) && (speed_trg <=C_SPEED_1KMPH)));

% Speed trg is 2km/h  or Prev_Speed is less than 1km/h

aVarTruthTableCondition_4 = logical((Prev_Speed ==  C_SPEED_1KMPH) && ((speed_trg == C_SPEED_2KMPH) || (speed_trg == C_SPEED_ZERO)));

% Prev_Speed is 1km/h and Speed trim is 0

aVarTruthTableCondition_5 = logical(((Prev_Speed ==  C_SPEED_1KMPH) && (speed_trim == C_SPEED_ZERO)));

% pre Speed is 0km/h and Other Conditions

aVarTruthTableCondition_6 = logical((Prev_Speed ==  C_SPEED_ZERO) && ((speed_trg == C_SPEED_2KMPH) || (speed_trg == C_SPEED_1KMPH)));

if (aVarTruthTableCondition_1)
    aFcnTruthTableAction_1();
elseif (aVarTruthTableCondition_2)
    aFcnTruthTableAction_2();
elseif (aVarTruthTableCondition_3)
    aFcnTruthTableAction_3();
elseif (aVarTruthTableCondition_4)
    aFcnTruthTableAction_1();
elseif (aVarTruthTableCondition_5)
    aFcnTruthTableAction_4();
elseif (aVarTruthTableCondition_6)
    aFcnTruthTableAction_1();
else % Default
    aFcnTruthTableAction_5();
end

function aFcnTruthTableAction_1()

% Update Speed_k with Speed trigger

Speed = speed_trg;

function aFcnTruthTableAction_2()

% Update Speed_k with 2km/h

Speed = C_SPEED_2KMPH;

function aFcnTruthTableAction_3()

% Update Speed_k with 1km/h

Speed = C_SPEED_1KMPH;

function aFcnTruthTableAction_4()

% Update Speed_k with 0km/h

Speed = C_SPEED_ZERO;

function aFcnTruthTableAction_5()

% No Change

Speed = Prev_Speed;
